simulink model "furuta_rl_balance_s2r"  (R2025a)
settings: Solver=VariableStepAuto  StartTime=0.0  StopTime=50  RelTol=1e-3
values from neighbouring files (symbols this model uses):
  al0 = 0.25 * (2*rand - 1)    [localResetFcn.m]    (also in s2l_rework.m = al0_rng   * (2*rand - 1))
  ald0 = 0.30 * (2*rand - 1)    [localResetFcn.m]    (also in s2l_rework.m = ald0_rng  * (2*rand - 1))
  p = getNominalPlantParams()    [s2l_rework.m]
  th0 = 0.15 * (2*rand - 1)    [localResetFcn.m]    (also in s2l_rework.m = th0_rng   * (2*rand - 1))
  th_ref0 = 0    [localResetFcn.m]    (also in s2l_rework.m = thref_rng * (2*rand - 1))
  thd0 = 0.20 * (2*rand - 1)    [localResetFcn.m]    (also in s2l_rework.m = thd0_rng  * (2*rand - 1))
libraries: rllib x1
settings Model: Creator=deng_zhiwen  LastModifiedBy=deng_zhiwen

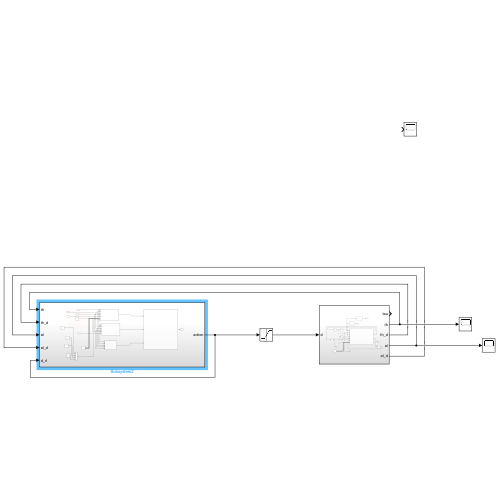
[thumbnail: Simulink's stored preview of the top-level diagram]
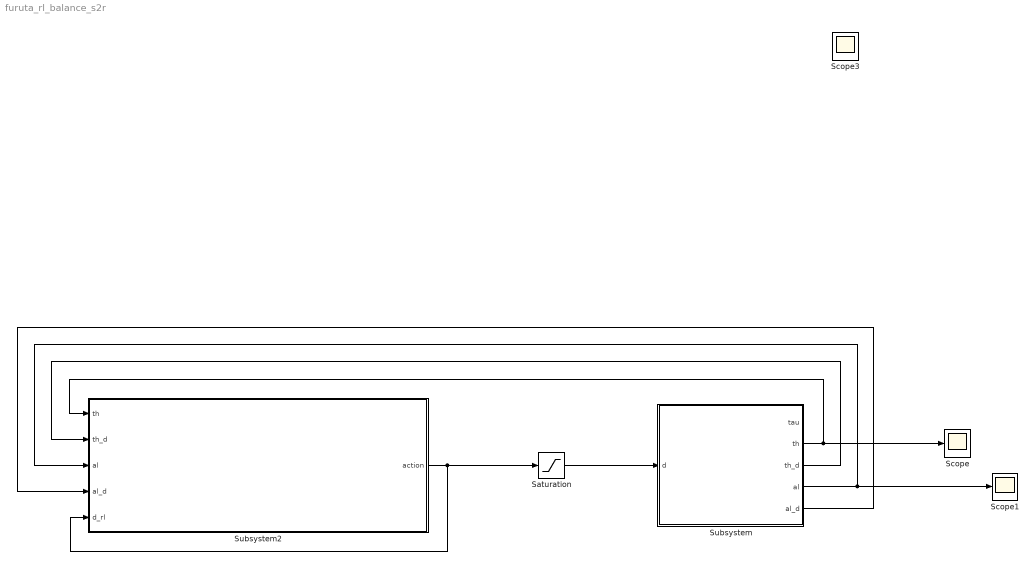
== system furuta_rl_balance_s2r ==
  Saturation : Saturate  UpperLimit=1  LowerLimit=-1
  Scope : Scope
      settings: ActiveDisplayYMinimum=-1  ActiveDisplayYMaximum=1
  Scope1 : Scope
      settings: ActiveDisplayYMinimum=-0.4013782374355474  ActiveDisplayYMaximum=0.32817211347176795
  Scope3 : Scope
      settings: ActiveDisplayYMinimum=-1  ActiveDisplayYMaximum=1  DataLoggingVariableName=ScopeData3
  Subsystem : Subsystem
  Subsystem2 : Subsystem
  wires:
  Subsystem/2(th) -> Scope/1, Subsystem2/1(th)
  Subsystem/3(th_d) -> Subsystem2/2(th_d)
  Subsystem/4(al) -> Scope1/1, Subsystem2/3(al)
  Subsystem/5(al_d) -> Subsystem2/4(al_d)
  Subsystem2/1(action) -> Saturation/1, Subsystem2/5(d_rl)
  Saturation/1 -> Subsystem/1(d)

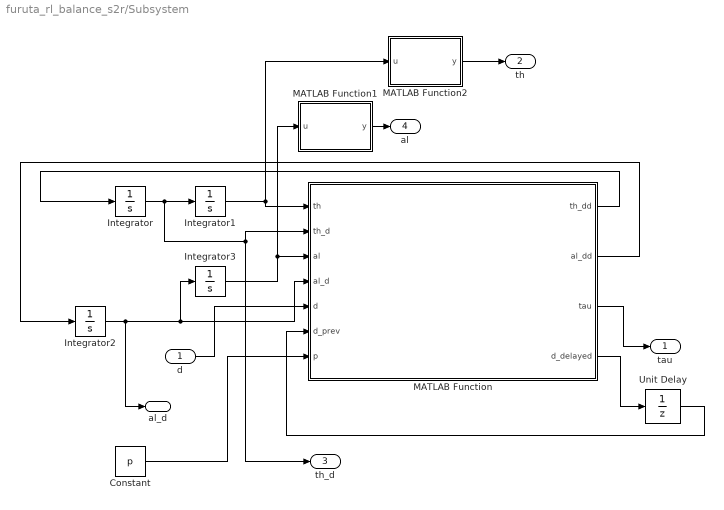
== system furuta_rl_balance_s2r/Subsystem ==
  d : Inport
  Constant : Constant  Value=p  OutDataTypeStr=Bus: PlantPBus
  Integrator : Integrator  InitialCondition=thd0
  Integrator1 : Integrator  InitialCondition=th0
  Integrator2 : Integrator  InitialCondition=ald0
  Integrator3 : Integrator  InitialCondition=al0
  MATLAB Function : MATLAB Function  TreatAsAtomicUnit=on
  MATLAB Function1 : MATLAB Function  TreatAsAtomicUnit=on
  MATLAB Function2 : MATLAB Function  TreatAsAtomicUnit=on
  Unit Delay : UnitDelay  SampleTime=-1  HasFrameUpgradeWarning=on
  tau : Outport
  th : Outport  Port=2
  th_d : Outport  Port=3
  al : Outport  Port=4
  al_d : Outport  Port=5
  wires:
  MATLAB Function/1(th_dd) -> Integrator/1
  MATLAB Function/2(al_dd) -> Integrator2/1
  Integrator/1 -> Integrator1/1, MATLAB Function/2(th_d), th_d/1
  d/1 -> MATLAB Function/5(d)
  Integrator2/1 -> MATLAB Function/4(al_d), Integrator3/1, al_d/1
  MATLAB Function/3(tau) -> tau/1
  Integrator1/1 -> MATLAB Function2/1(u), MATLAB Function/1(th)
  Integrator3/1 -> MATLAB Function1/1(u), MATLAB Function/3(al)
  MATLAB Function1/1(y) -> al/1
  MATLAB Function2/1(y) -> th/1
  Constant/1 -> MATLAB Function/7(p)
  MATLAB Function/4(d_delayed) -> Unit Delay/1
  Unit Delay/1 -> MATLAB Function/6(d_prev)

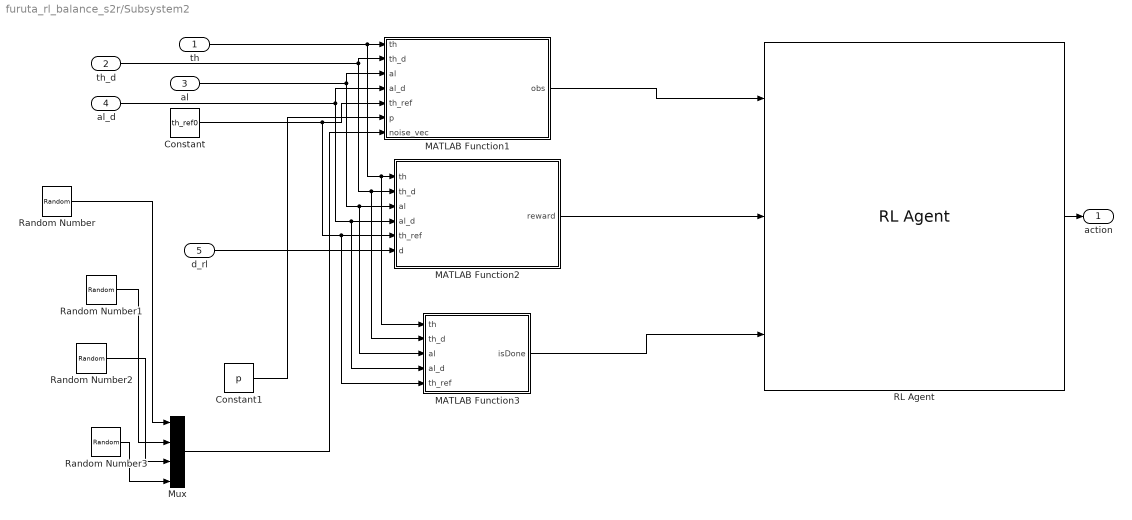
== system furuta_rl_balance_s2r/Subsystem2 ==
  th : Inport
  th_d : Inport  Port=2
  al : Inport  Port=3
  al_d : Inport  Port=4
  d_rl : Inport  Port=5
  Constant : Constant  Value=th_ref0
  Constant1 : Constant  Value=p  OutDataTypeStr=Bus: PlantPBus
  MATLAB Function1 : MATLAB Function  TreatAsAtomicUnit=on
  MATLAB Function2 : MATLAB Function  TreatAsAtomicUnit=on
  MATLAB Function3 : MATLAB Function  TreatAsAtomicUnit=on
  Mux : Mux
  RL Agent : rllib/RL Agent  Agent=agent  ExternalActionAsInput=off  ProvideLastAction=off  ProvideCumRwd=off  TreatAsDirectFeedthrough=on  UseStrictObservationDataTypes=off
  Random Number{,1..3} (4 alike) : RandomNumber  SampleTime=0.01
  action : Outport
  wires:
  al/1 -> MATLAB Function2/3(al), MATLAB Function3/3(al), MATLAB Function1/3(al)
  th/1 -> MATLAB Function3/1(th), MATLAB Function2/1(th), MATLAB Function1/1(th)
  MATLAB Function2/1(reward) -> RL Agent/2
  MATLAB Function1/1(obs) -> RL Agent/1
  al_d/1 -> MATLAB Function2/4(al_d), MATLAB Function3/4(al_d), MATLAB Function1/4(al_d)
  th_d/1 -> MATLAB Function2/2(th_d), MATLAB Function3/2(th_d), MATLAB Function1/2(th_d)
  d_rl/1 -> MATLAB Function2/6(d)
  RL Agent/1 -> action/1
  Constant/1 -> MATLAB Function2/5(th_ref), MATLAB Function3/5(th_ref), MATLAB Function1/5(th_ref)
  MATLAB Function3/1(isDone) -> RL Agent/3
  Constant1/1 -> MATLAB Function1/6(p)
  Random Number/1 -> Mux/1
  Random Number1/1 -> Mux/2
  Random Number2/1 -> Mux/3
  Random Number3/1 -> Mux/4
  Mux/1 -> MATLAB Function1/7(noise_vec)

== matlab function furuta_rl_balance_s2r/Subsystem/MATLAB Function1 ==
  data: u input; y output
function y = wrap_angle(u)
    y = atan2(sin(u), cos(u));
end

== matlab function furuta_rl_balance_s2r/Subsystem/MATLAB Function ==
  data: th input; th_dd output size=1; th_d input; al input; al_d input; d input; d_prev input; al_dd output size=1; tau output size=1; p input; d_delayed output
function [th_dd, al_dd, tau, d_delayed] = furuta_step_sim2real(th, th_d, al, al_d, d, d_prev, p)
%#codegen
% 相比原版新增：
% 1) d_prev：上一步实际执行的动作（用于模拟执行器一阶延迟）
% 2) d_delayed：本步实际执行动作（输出，供下一步使用）
% 3) dist_th / dist_al 确保被使用

% -------------------------------------------------------------------------
% 1) 参数读取
% -------------------------------------------------------------------------
J_theta = p.J_theta;
J_alpha = p.J_alpha;
m_p     = p.m_p;
r       = p.r;
l       = p.l;
g_val   = p.g;

B_r     = p.B_r;
B_p     = p.B_p;

K_g     = p.K_g;
V_s     = p.V_s;
R_m     = p.R_m;
k_t     = p.k_t;
k_e     = p.k_e;
eta_m   = p.eta_m;
eta_g   = p.eta_g;
tau_max = p.tau_max;

deadzone   = p.deadzone;
tau_offset = p.tau_offset;
Fc_r       = p.Fc_r;
Fc_p       = p.Fc_p;
w_eps      = max(p.w_eps, 1e-3);

dist_th = p.dist_th;
dist_al = p.dist_al;

% -------------------------------------------------------------------------
% 2) 执行器一阶延迟
%    模拟电机+驱动器响应延迟
%    alpha_act 越小 = 延迟越大
%    alpha_act = 1.0 表示无延迟（原始行为）
%    alpha_act = 0.6 表示约一步半的等效延迟
% -------------------------------------------------------------------------
alpha_act = p.alpha_act;   % 从参数结构体读取，方便随机化
d_delayed = alpha_act * d + (1.0 - alpha_act) * d_prev;

% -------------------------------------------------------------------------
% 3) 动作限幅 + 死区（作用在延迟后的动作上）
% -------------------------------------------------------------------------
d_use = max(-1.0, min(1.0, d_delayed));

if abs(d_use) < deadzone
    d_eff = 0.0;
else
    d_eff = sign(d_use) * (abs(d_use) - deadzone) / (1.0 - deadzone);
end

% -------------------------------------------------------------------------
% 4) 电机模型
% -------------------------------------------------------------------------
Cd = eta_m * eta_g * K_g * k_t * V_s / R_m;
Cv = eta_m * eta_g * K_g^2 * k_t * k_e / R_m;

tau_raw = Cd * d_eff - Cv * th_d + tau_offset;
tau     = max(-tau_max, min(tau_max, tau_raw));

% -------------------------------------------------------------------------
% 5) 等效动力学参数
% -------------------------------------------------------------------------
a  = J_theta + m_p * r^2;
c  = J_alpha + m_p * l^2;
e  = m_p * r * l;
g0 = m_p * g_val * l;
b  = e * cos(al);

% -------------------------------------------------------------------------
% 6) 平滑库仑摩擦
% -------------------------------------------------------------------------
fr = Fc_r * tanh(th_d / w_eps);
fp = Fc_p * tanh(al_d / w_eps);

% -------------------------------------------------------------------------
% 7) 右端项（含外部扰动）
% -------------------------------------------------------------------------
rhs1 = tau          ...
     - B_r * th_d   ...
     - fr            ...
     + e * sin(al) * al_d^2 ...
     + dist_th;

rhs2 = - B_p * al_d ...
     - fp            ...
     + g0 * sin(al)  ...
     + dist_al;

% -------------------------------------------------------------------------
% 8) 求解加速度
% -------------------------------------------------------------------------
detM = a * c - b^2;
detM = max(detM, 1e-8);

th_dd = ( c * rhs1 - b * rhs2) / detM;
al_dd = (-b * rhs1 + a * rhs2) / detM;

end

== matlab function furuta_rl_balance_s2r/Subsystem/MATLAB Function2 ==
  data: u input; y output
function y = wrap_angle(u)
    y = atan2(sin(u), cos(u));
end

== matlab function furuta_rl_balance_s2r/Subsystem2/MATLAB Function1 ==
  data: th input; obs output; th_d input; al input; al_d input; th_ref input; p input; noise_vec input
function obs = obs_builder(th, th_d, al, al_d, th_ref, p, noise_vec)
%#codegen
% noise_vec: [n_th; n_thd; n_al; n_ald]，由外部Random Number模块生成

% -------------------------------------------------------------------------
% 1) 读取噪声
% -------------------------------------------------------------------------
n_th  = 0.0;
n_thd = 0.0;
n_al  = 0.0;
n_ald = 0.0;

if isfield(p, 'noise_th_std')
    n_th  = p.noise_th_std  * noise_vec(1);
    n_thd = p.noise_thd_std * noise_vec(2);
    n_al  = p.noise_al_std  * noise_vec(3);
    n_ald = p.noise_ald_std * noise_vec(4);
end

% -------------------------------------------------------------------------
% 2) 加噪声后的传感器读数
% -------------------------------------------------------------------------
th_noisy   = th   + n_th;
th_d_noisy = th_d + n_thd;
al_noisy   = al   + n_al;
al_d_noisy = al_d + n_ald;

% -------------------------------------------------------------------------
% 3) 构造观测
% -------------------------------------------------------------------------
e_th = th_noisy - th_ref;

obs = zeros(5, 1);
obs(1) = e_th;
obs(2) = th_d_noisy;
obs(3) = cos(al_noisy);
obs(4) = sin(al_noisy);
obs(5) = al_d_noisy;

end

== matlab function furuta_rl_balance_s2r/Subsystem2/MATLAB Function2 ==
  data: th input; reward output; th_d input; al input; al_d input; th_ref input; d input
function reward = reward_builder(th, th_d, al, al_d, th_ref, d)
%#codegen
% 奖励函数（平滑稳健版）
%
% 目标：
% 1) 保持摆杆 al = 0 附近（倒立）
% 2) 旋转臂 th 跟踪 th_ref
% 3) 抑制速度过大
% 4) 抑制控制输入过大

e_th = th - th_ref;
e_al = wrap_angle(al);

% -----------------------------
% 权重参数（建议先从这组开始）
% -----------------------------
w_al  = 8.0;     % 摆杆角度误差权重（主目标）
w_th  = 1.0;     % 旋转臂位置误差权重
%w_ald = 0.3;     % 摆杆角速度权重
w_ald = 0.8;
%w_thd = 0.05;    % 旋转臂角速度权重
w_thd = 0.15;    % 旋转臂角速度权重
%w_u   = 0.001;   % 控制输入权重
w_u   = 0.003;   % 控制输入权重

% -----------------------------
% 基础奖励
% -----------------------------
reward = 1.0;

% -----------------------------
% 平滑惩罚项
% -----------------------------
reward = reward ...
    - w_al  * (e_al^2) ...
    - w_th  * (e_th^2) ...
    - w_ald * (al_d^2) ...
    - w_thd * (th_d^2) ...
    - w_u   * (d^2);

% -----------------------------
% 小范围稳态奖励
% -----------------------------
if abs(e_al) < 8*pi/180
    reward = reward + 0.5;
end

if abs(e_al) < 5*pi/180 && abs(e_th) < 8*pi/180
    reward = reward + 0.5;
end

if abs(e_al) < 5*pi/180 && abs(al_d) < 0.5 ...
        && abs(e_th) < 8*pi/180 && abs(th_d) < 0.5
    reward = reward + 1.0;
end

% -----------------------------
% 接近失稳时附加惩罚
% -----------------------------
if abs(e_al) > 20*pi/180
    reward = reward - 5.0;
end

end

function y = wrap_angle(u)
y = mod(u + pi, 2*pi) - pi;
end

== matlab function furuta_rl_balance_s2r/Subsystem2/MATLAB Function3 ==
  data: th input; isDone output; th_d input; al input; al_d input; th_ref input
function isDone = isdone_builder(th, th_d, al, al_d, th_ref)
%#codegen
% episode终止逻辑
%
% 训练目标：
% 1) 倒立平衡
% 2) 旋转臂不要偏离参考太远
% 3) 速度不要发散

e_th = th - th_ref;
e_al = wrap_angle(al);

isDone = false;

% 1) 摆杆偏离过大：平衡失败
if abs(e_al) > 30*pi/180
    isDone = true;
    return;
end

% 2) 旋转臂偏离参考过大
if abs(e_th) > 0.8
    isDone = true;
    return;
end

% 3) 速度过大：认为系统发散
if abs(al_d) > 20
    isDone = true;
    return;
end

if abs(th_d) > 20
    isDone = true;
    return;
end

end

function y = wrap_angle(u)
y = mod(u + pi, 2*pi) - pi;
end
